simulink library "RotationalDynamics"  (R2015a)
settings: Solver=ode45  StartTime=0.0  StopTime=10.0  RelTol=1e-3
undefined symbols (not defined in the file or in its folder): I
libraries: lib_gravity x2, aerolibutil x1, aerolibtransform2 x1
settings Model: Creator=bbrito  LastModifiedBy=bbrito

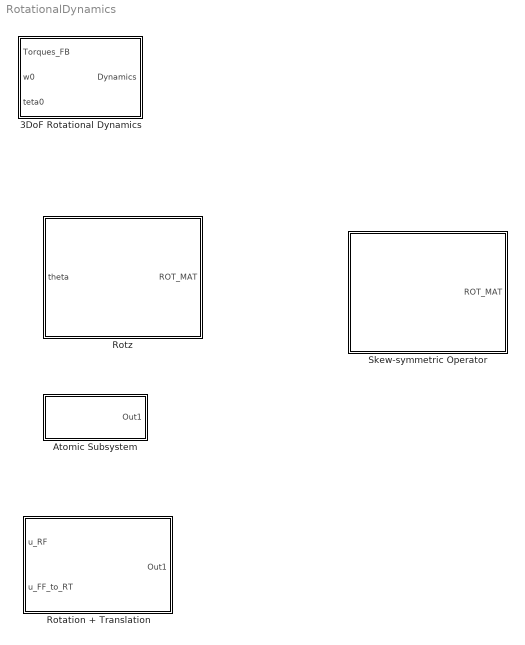
== system RotationalDynamics ==
  3DoF Rotational Dynamics : Subsystem  TreatAsAtomicUnit=on  mask{I=I}
      mask prompts: I "Inertia"
  Atomic Subsystem : Subsystem  TreatAsAtomicUnit=on  mask{omega=[0;0;0], offset=0}
      mask prompts: omega "Rotation Vector rad/s"; offset "Offset rad"
  Rotation + Translation : Subsystem  TreatAsAtomicUnit=on
  Rotz : Subsystem  TreatAsAtomicUnit=on
      mask help:
      | ESA-ESTEC
      | ---------------------------------------------------------------------------
      | Version:0.0          Date:2010/20015          Author: #BB
      | Matlab version: 2015a          Project: AIM          Division: TEC-ECN
      | ---------------------------------------------------------------------------
      | This block models z axis rotation matrix.
      |
      | The input is the z rotation angle.
  Skew-symmetric Operator : Subsystem  AncestorBlock=RotationalDynamics/Rotz  TreatAsAtomicUnit=on  mask{omega=[0;0;0]}
      mask prompts: omega "Rotation Speed Vector [wx wy wz] rad/s"
      mask help:
      | ESA-ESTEC
      | ---------------------------------------------------------------------------
      | Version:0.0          Date:08/11/20015          Author: #BB
      | Matlab version: 2015a          Project: AIM          Division: TEC-ECN
      | ---------------------------------------------------------------------------
      | This block models a Skew-symmetrix matrix.
      |
      | The input is the wx,wy,wz relative angular velocity in rad/s.

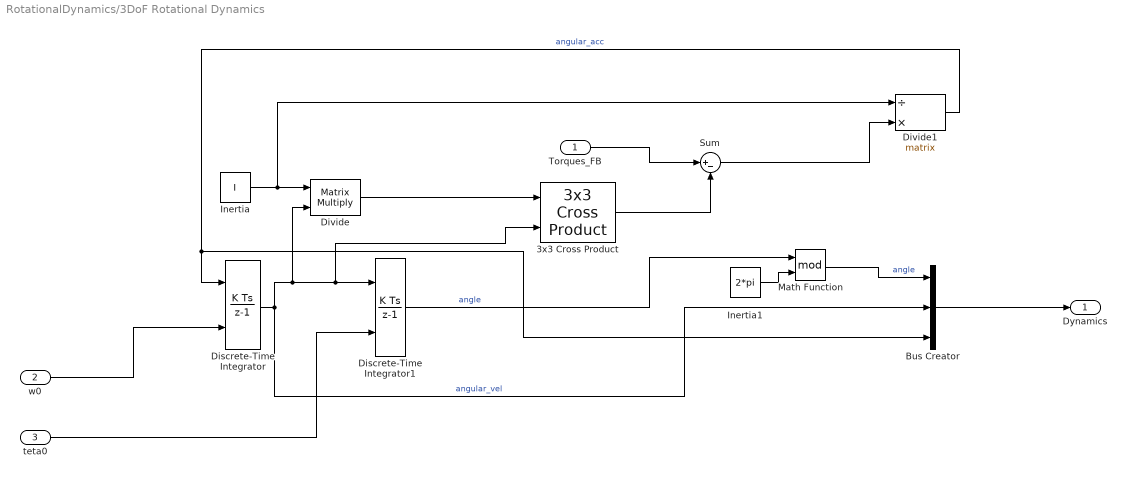
== system RotationalDynamics/3DoF Rotational Dynamics ==
  Torques_FB : Inport
  w0 : Inport  Port=2
  teta0 : Inport  Port=3
  3x3 Cross Product : aerolibutil/3x3 Cross Product
  Bus Creator : BusCreator  Inputs=3
  Discrete-Time Integrator : DiscreteIntegrator  InitialConditionSource=external  InitialConditionSetting=State (most efficient)
  Discrete-Time Integrator1 : DiscreteIntegrator  InitialConditionSource=external  InitialConditionSetting=State (most efficient)
  Divide : Product  Inputs=**  Multiplication=Matrix(*)
  Divide1 : Product  Inputs=/*  Multiplication=Matrix(*)
  Inertia : Constant  Value=I
  Inertia1 : Constant  Value=2*pi
  Math Function : Math  Operator=mod  SaturateOnIntegerOverflow=on
  Sum : Sum  Inputs=|+-
  Dynamics : Outport
  wires:
  Discrete-Time Integrator/1 -> Bus Creator/2, Divide/2, 3x3 Cross Product/2, Discrete-Time Integrator1/1  "angular_vel"
  teta0/1 -> Discrete-Time Integrator1/2
  w0/1 -> Discrete-Time Integrator/2
  Inertia/1 -> Divide1/1, Divide/1
  Divide/1 -> 3x3 Cross Product/1
  Torques_FB/1 -> Sum/1
  3x3 Cross Product/1 -> Sum/2
  Sum/1 -> Divide1/2
  Divide1/1 -> Discrete-Time Integrator/1, Bus Creator/3  "angular_acc"
  Bus Creator/1 -> Dynamics/1
  Inertia1/1 -> Math Function/2
  Discrete-Time Integrator1/1 -> Math Function/1  "angle"
  Math Function/1 -> Bus Creator/1  "angle"

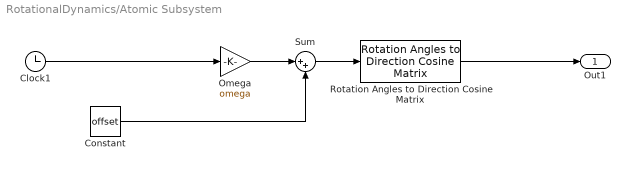
== system RotationalDynamics/Atomic Subsystem ==
  Clock1 : Clock
  Constant : Constant  Value=offset
  Omega : Gain  Gain=omega
  Rotation Angles to Direction Cosine Matrix : aerolibtransform2/Rotation Angles to Direction Cosine Matrix  rotationOrder=XYZ
  Sum : Sum  Inputs=|++
  Out1 : Outport
  wires:
  Rotation Angles to Direction Cosine Matrix/1 -> Out1/1
  Omega/1 -> Sum/1
  Clock1/1 -> Omega/1
  Constant/1 -> Sum/2
  Sum/1 -> Rotation Angles to Direction Cosine Matrix/1

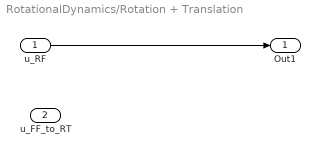
== system RotationalDynamics/Rotation + Translation ==
  u_RF : Inport
  u_FF_to_RT : Inport  Port=2
  Out1 : Outport
  wires:
  u_RF/1 -> Out1/1

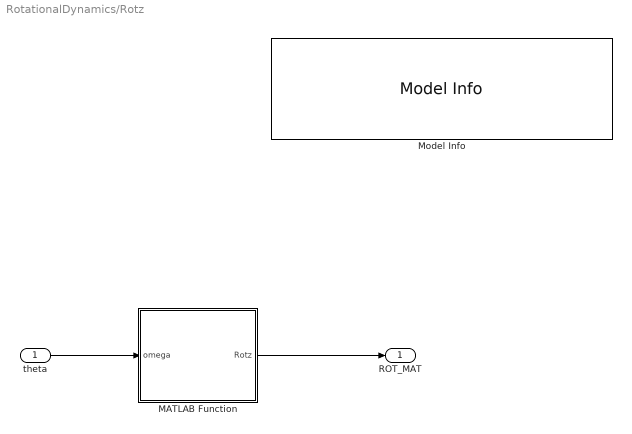
== system RotationalDynamics/Rotz ==
  theta : Inport
  MATLAB Function : MATLAB Function  TreatAsAtomicUnit=on
  Model Info : lib_gravity/Spherical Gravity Acceleration/Model Info  Frame=on  DisplayStringWithTags=|  HorizontalTextAlignment=Center  LeftAlignmentValue=0.5  SourceBlockDiagram=RotationalDynamics  TagMaxNumber=20
      | ESA-ESTEC
      | ---------------------------------------------------------------------------
      | Version:0.0          Date:2010/20015          Author: #BB
      | Matlab version: 2015a          Project: AIM          Division: TEC-ECN
      | ---------------------------------------------------------------------------
      | This block models a body constant rotation.
      | 
      | The input is the x,y,z relative to the center of mass of the body.
  ROT_MAT : Outport
  wires:
  MATLAB Function/1(Rotz) -> ROT_MAT/1
  theta/1 -> MATLAB Function/1(omega)

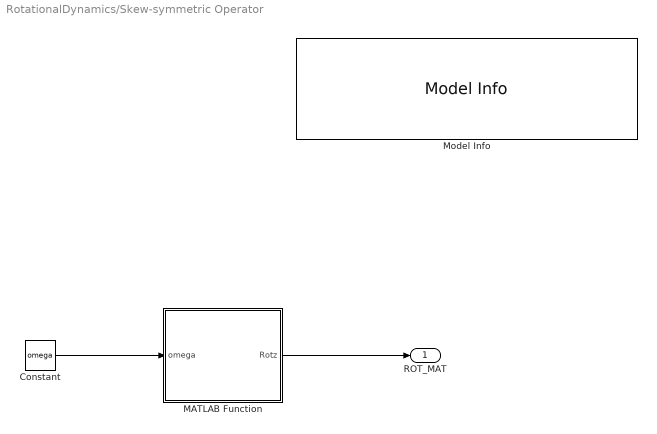
== system RotationalDynamics/Skew-symmetric Operator ==
  Constant : Constant  Value=omega
  MATLAB Function : MATLAB Function  TreatAsAtomicUnit=on
  Model Info : lib_gravity/Spherical Gravity Acceleration/Model Info  Frame=on  DisplayStringWithTags=|  HorizontalTextAlignment=Center  LeftAlignmentValue=0.5  SourceBlockDiagram=RotationalDynamics  TagMaxNumber=20
      | ESA-ESTEC
      | ---------------------------------------------------------------------------
      | Version:0.0          Date:2010/20015          Author: #BB
      | Matlab version: 2015a          Project: AIM          Division: TEC-ECN
      | ---------------------------------------------------------------------------
      | This block models a body constant rotation.
      | 
      | The input is the x,y,z relative to the center of mass of the body.
  ROT_MAT : Outport
  wires:
  MATLAB Function/1(Rotz) -> ROT_MAT/1
  Constant/1 -> MATLAB Function/1(omega)

== matlab function RotationalDynamics/Skew-symmetric Operator/MATLAB Function ==
  data: omega input; Rotz output
function Rotz = fcn(omega)

wx=omega(1);
wy=omega(2);
wz=omega(3);

H=[0 -wz wy;wz 0 -wx;-wy wx 0];

Rotz = H;

== matlab function RotationalDynamics/Rotz/MATLAB Function ==
  data: omega input; Rotz output
function Rotz = fcn(omega)

w=omega(3);

H=[cos(w) -sin(w) 0;sin(w) cos(w) 0;0 0 1];

Rotz = H;
